simulink model "DCMotorOLDCDC"  (R2018b)
settings: Solver=ode23tb  StartTime=0.0  StopTime=15  MaxStep=1e-4  MinStep=1e-5  RelTol=1e-2
libraries: powerlib x31, powerlib_meascontrol x1
settings Model: Creator=Koosha  LastModifiedBy=Koosha
settings SolverCC: ZeroCrossAlgorithm=Adaptive
settings DebuggingCC: IgnoredZcDiagnostic=none

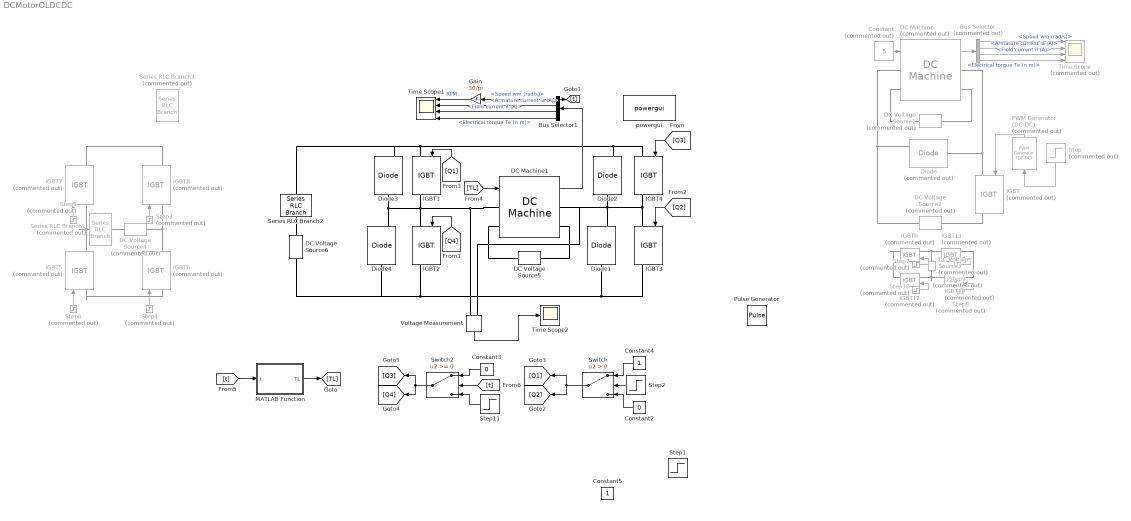
== system DCMotorOLDCDC ==
  Bus Selector : BusSelector  Commented=on  OutputSignals=Speed wm (rad/s),Armature current ia (A),Field current if (A),Electrical torque Te (n m)
  Bus Selector1 : BusSelector  OutputSignals=Speed wm (rad/s),Armature current ia (A),Field current if (A),Electrical torque Te (n m)
  Constant : Constant  Commented=on  Value=5
  Constant2 : Constant  Value=0
  Constant3 : Constant  Value=0
  Constant4 : Constant
  Constant5 : Constant
  DC Machine : powerlib/Machines/DC Machine  Commented=on  PresetModel=03: 5HP 500V 1750RPM Field:300V  MechanicalLoad=Torque TL  FieldType=Wound  ShowDetailedParameters=on  MeasurementBus=off  RLa=[11.2 0.1215]  RLf=[281.3 156]  Laf=1.976  MachineConstant=Torque constant (N.m/A)  Ke=1.8  Kt=1.8  J=0.02215  Bm=0.002953  Tf=0.5161  w0=0  Ifinit=0  TsPowergui=0  TsBlock=-1
  DC Machine1 : powerlib/Machines/DC Machine  PresetModel=03: 5HP 500V 1750RPM Field:300V  MechanicalLoad=Torque TL  FieldType=Wound  ShowDetailedParameters=on  MeasurementBus=off  RLa=[11.2 0.1215]  RLf=[281.3 156]  Laf=1.976  MachineConstant=Torque constant (N.m/A)  Ke=1.8  Kt=1.8  J=0.02215  Bm=0.002953  Tf=0.5161  w0=0  Ifinit=0  TsPowergui=0  TsBlock=-1
  DC Voltage Source1 : powerlib/Electrical Sources/DC Voltage Source  Commented=on  Amplitude=300  Measurements=None
  DC Voltage Source2 : powerlib/Electrical Sources/DC Voltage Source  Commented=on  Amplitude=500  Measurements=None
  DC Voltage Source3 : powerlib/Electrical Sources/DC Voltage Source  Commented=on  Amplitude=300  Measurements=None
  DC Voltage Source4 : powerlib/Electrical Sources/DC Voltage Source  Commented=on  Amplitude=500  Measurements=None
  DC Voltage Source5 : powerlib/Electrical Sources/DC Voltage Source  Amplitude=300  Measurements=None
  DC Voltage Source6 : powerlib/Electrical Sources/DC Voltage Source  Amplitude=500  Measurements=None
  Diode : powerlib/Power Electronics/Diode  Commented=on  Ron=0.001  Lon=0  Vf=0.8  IC=0  UseSnubber=0  Rs=500  Cs=250e-9  Measurements=on
  Diode{1..4} (4 alike) : powerlib/Power Electronics/Diode  Ron=0.001  Lon=0  Vf=0.8  IC=0  UseSnubber=0  Rs=inf  Cs=inf  Measurements=on
  Gain : Gain  Gain=30/pi
  IGBT{,5..12} (9 alike) : powerlib/Power Electronics/IGBT  Commented=on  Ron=0.001  Lon=0  Vf=1  Tf=1e-6  Tt=2e-6  IC=0  Rs=1e5  Cs=inf  Measurements=on
  IGBT{1..4} (4 alike) : powerlib/Power Electronics/IGBT  Ron=0.001  Lon=0  Vf=1  Tf=1e-6  Tt=2e-6  IC=0  Rs=1e6  Cs=1e-6  Measurements=on
  MATLAB Function : MATLAB Function  TreatAsAtomicUnit=on
  PWM Generator (DC-DC) : powerlib_meascontrol/Pulse & Signal Generators/PWM Generator (DC-DC)  Commented=on  Fsw=5000  Ts=0
  Pulse Generator : DiscretePulseGenerator  PulseType=Time based  Period=2e-2  PulseWidth=50
  Series RLC Branch1 : powerlib/Elements/Series RLC Branch  Commented=on  LConnTagsString=__new0  RConnTagsString=__new0  BranchType=R  Resistance=100  Inductance=0  SetiL0=off  InitialCurrent=0  Capacitance=1e-6  Setx0=off  InitialVoltage=0  Measurements=None
  Series RLC Branch2 : powerlib/Elements/Series RLC Branch  LConnTagsString=__new0  RConnTagsString=__new0  BranchType=R  Resistance=100  Inductance=0  SetiL0=off  InitialCurrent=0  Capacitance=1e-6  Setx0=off  InitialVoltage=0  Measurements=None
  Series RLC Branch3 : powerlib/Elements/Series RLC Branch  Commented=on  LConnTagsString=__new0  RConnTagsString=__new0  BranchType=L  Resistance=100  Inductance=1e-6  SetiL0=off  InitialCurrent=0  Capacitance=1e-6  Setx0=off  InitialVoltage=0  Measurements=None
  Step : Step  Commented=on  Time=0.5  Before=0.2  After=0.8  SampleTime=0
  Step1 : Step  Time=12  SampleTime=0
  Step10 : Step  Commented=on  Time=0.5  Before=1  After=0  SampleTime=0
  Step11 : Step  Time=12  Before=1  After=0  SampleTime=0
  Step2 : Step  Time=5  Before=1  After=0  SampleTime=0
  Step3 : Step  Commented=on  Time=5  SampleTime=0
  Step4 : Step  Commented=on  Time=5  Before=1  After=0  SampleTime=0
  Step5 : Step  Commented=on  Time=5  Before=1  After=0  SampleTime=0
  Step6 : Step  Commented=on  Time=5  SampleTime=0
  Step7 : Step  Commented=on  Time=0.5  SampleTime=0
  Step8 : Step  Commented=on  Time=0.5  SampleTime=0
  Step9 : Step  Commented=on  Time=0.5  Before=1  After=0  SampleTime=0
  Switch : Switch  Criteria=u2 > Threshold
  Switch2 : Switch
  Time Scope : Scope  Commented=on  NumInputPorts=4
  Time Scope1 : Scope  NumInputPorts=4
  Time Scope2 : Scope
  Voltage Measurement : powerlib/Measurements/Voltage Measurement  PhasorSimulation=off  OutputType=Complex  PSBequivalent=0
  powergui : powerlib/powergui  Priority=1  SimulationMode=Discrete  SampleTime=5e-5  frequency=60  Iterations=50  frequencyindice=0  Pbase=100e6  ErrMax=1e-4  UnitsV=kV  UnitsW=MW  buscounter=0  FunctionMessages=off  echomessages=off  EnableUseOfTLC=off  CurrentSourceSwitches=off  DisableSnubberDevices=off  DisableRonSwitches=off  DisableVfSwitches=off  DisplayEquations=off  SolverType=Tustin/Backward Euler (TBE)  Interpol=off  ExternalGateDelay=off  methode=off  Ts=100  x0status=blocks  SPID=on  SwTol=0  HookPort=off  RestoreLinks=warning  ResistiveCurrentMeasurement=off  Frange=[0:2:500]  Ylog=off  Xlog=on  ShowGrid=off  save=off  variable=ZData  structure=0  ZoomFFT=off  StartTime=0.0  cycles=1  DisplayStyle=1  fundamental=60  FreqAxis=off  MaxFrequency=1000  frequencyindicesteady=1  RmsSteady=1  display=off
  wires:
  Constant/1 -> DC Machine/1
  PWM Generator (DC-DC)/1 -> IGBT/1
  Step/1 -> PWM Generator (DC-DC)/1
  DC Machine/1 -> Bus Selector/1
  Bus Selector/1 -> Time Scope/1  "<Speed wm (rad/s)>"
  Bus Selector/2 -> Time Scope/2  "<Armature current ia (A)>"
  Bus Selector/3 -> Time Scope/3  "<Field current if (A)>"
  Bus Selector/4 -> Time Scope/4  "<Electrical torque Te (n m)>"
  Bus Selector1/3 -> Time Scope1/3  "<Field current if (A)>"
  Bus Selector1/2 -> Time Scope1/2  "<Armature current ia (A)>"
  DC Machine1/1 -> Bus Selector1/1
  Bus Selector1/4 -> Time Scope1/4  "<Electrical torque Te (n m)>"
  [Q1] -> IGBT1/1
  [Q2] -> IGBT3/1
  [Q4] -> IGBT2/1
  [Q3] -> IGBT4/1
  Constant2/1 -> Switch/3
  Step6/1 -> IGBT5/1
  Step3/1 -> IGBT8/1
  Step4/1 -> IGBT6/1
  Step5/1 -> IGBT7/1
  Step7/1 -> IGBT9/1
  Step8/1 -> IGBT10/1
  Step9/1 -> IGBT11/1
  Step10/1 -> IGBT12/1
  Gain/1 -> Time Scope1/1  "RPM"
  Bus Selector1/1 -> Gain/1, [t]  "<Speed wm (rad/s)>"
  Voltage Measurement/1 -> Time Scope2/1
  Constant4/1 -> Switch/1
  MATLAB Function/1(TL) -> [TL]
  [t] -> MATLAB Function/1(t)
  [TL] -> DC Machine1/1
  Switch/1 -> [Q2], [Q1]
  Step2/1 -> Switch/2
  Switch2/1 -> [Q4], [Q3]
  Constant3/1 -> Switch2/1
  Step11/1 -> Switch2/3
  [t] -> Switch2/2
  connections:
  IGBT/RConn1 -- DC Voltage Source2/LConn1
  DC Voltage Source1/RConn1 -- DC Machine/LConn2
  DC Voltage Source1/LConn1 -- DC Machine/RConn2
  DC Voltage Source2/RConn1 -- Diode/RConn1 -- DC Machine/LConn1
  IGBT/LConn1 -- Diode/LConn1 -- DC Machine/RConn1
  IGBT3/LConn1 -- Voltage Measurement/LConn2 -- DC Machine1/RConn1 -- Diode2/LConn1 -- Diode1/RConn1 -- IGBT4/RConn1
  Series RLC Branch2/RConn1 -- Diode3/RConn1 -- IGBT1/LConn1 -- IGBT4/LConn1 -- Diode2/RConn1
  IGBT5/LConn1 -- IGBT6/LConn1
  IGBT6/RConn1 -- DC Voltage Source4/LConn1 -- IGBT8/LConn1
  Series RLC Branch1/RConn1 -- IGBT7/LConn1 -- IGBT5/RConn1
  IGBT11/RConn1 -- DC Voltage Source3/LConn1 -- IGBT9/LConn1
  IGBT9/RConn1 -- IGBT12/RConn1
  IGBT10/RConn1 -- DC Voltage Source3/RConn1 -- IGBT12/LConn1
  IGBT11/LConn1 -- IGBT10/LConn1
  Series RLC Branch1/LConn1 -- DC Voltage Source4/RConn1
  IGBT2/RConn1 -- DC Voltage Source6/LConn1 -- Diode4/LConn1 -- Diode1/LConn1 -- IGBT3/RConn1
  IGBT7/RConn1 -- IGBT8/RConn1
  Series RLC Branch2/LConn1 -- DC Voltage Source6/RConn1
  DC Voltage Source5/LConn1 -- DC Machine1/RConn2
  DC Machine1/LConn2 -- DC Voltage Source5/RConn1
  Diode3/LConn1 -- IGBT1/RConn1 -- Voltage Measurement/LConn1 -- DC Machine1/LConn1 -- IGBT2/LConn1 -- Diode4/RConn1

== matlab function DCMotorOLDCDC/MATLAB Function ==
  data: t input; TL output
function TL = fcn(t)

 if t == 0
     TL = 0
 elseif t>0
     TL = 1
 elseif t<0   
     TL = -1
 else
     TL = 1
 end
end
